simulink model "SimpleImpedance_Main"  (R2016b)
settings: Solver=VariableStepAuto  StartTime=0.0  StopTime=30  RelTol=1e-3  EnableMultiTasking=on
undefined symbols (not defined in the file): b, bh, C, dt, J, Jh, JJ, k, K, K_f, Ke, kh, M
settings Model: Creator=Minsu  LastModifiedBy=Minsu
settings DataIOCC: LimitDataPoints=on
settings OptimizationCC: LifeSpan=inf
settings DebuggingCC: AllowSymbolicDim=off  SFUnexpectedBacktrackingDiag=warning  SFNoUnconditionalDefaultTransitionDiag=warning  SFExecutionAtInitializationDiag=none
settings ModelReferenceCC: PropagateSignalLabelsOutOfModel=off
settings GRTTargetCC: TargetLangStandard=C89/C90 (ANSI)
settings ConfigComp: CovMetricSettings=dw  CovHtmlReporting=on  CovSaveCumulativeToWorkspaceVar=on  CovSaveSingleToWorkspaceVar=on  CovExternalEMLEnable=off

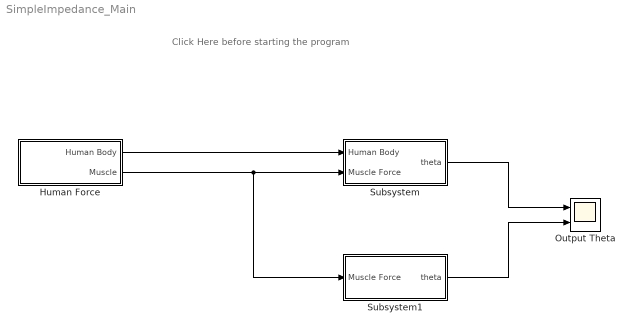
== system SimpleImpedance_Main ==
  note: Click Here before starting the program
  "Human Force " : Subsystem
  Output Theta : Scope  NumInputPorts=2
  Subsystem : Subsystem
  Subsystem1 : Subsystem
  wires:
  "Human Force "/1(Human Body) -> Subsystem/1(Human Body)
  "Human Force "/2(Muscle) -> Subsystem1/1(Muscle Force), Subsystem/2(Muscle Force)
  Subsystem/1(theta) -> Output Theta/1
  Subsystem1/1(theta) -> Output Theta/2

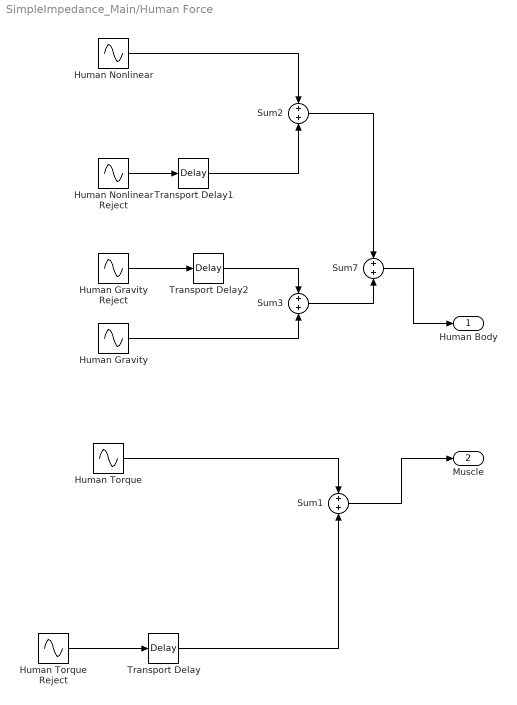
== system SimpleImpedance_Main/Human Force  ==
  Human Gravity : Sin  Amplitude=2  Frequency=2*pi*0.13  Phase=-30*pi/180
  Human Gravity Reject : Sin  Amplitude=-2  Frequency=2*pi*0.13  Phase=-30*pi/180
  Human Nonlinear : Sin  Amplitude=2.1  Frequency=2*pi*1.2
  Human Nonlinear Reject : Sin  Amplitude=-2.1  Frequency=2*pi*1.2
  Human Torque : Sin  Amplitude=10  Frequency=2*JJ*pi
  Human Torque Reject : Sin  Amplitude=-10  Frequency=JJ*2*pi
  Sum{1..3,7} (4 alike) : Sum
  Transport Delay : TransportDelay  DelayTime=3*1/JJ
  Transport Delay1 : TransportDelay  DelayTime=19*1/1.2
  Transport Delay2 : TransportDelay  DelayTime=12*1/0.13
  Human Body : Outport
  Muscle : Outport  Port=2
  wires:
  Sum7/1 -> Human Body/1
  Human Torque Reject/1 -> Transport Delay/1
  Human Torque/1 -> Sum1/1
  Sum1/1 -> Muscle/1
  Transport Delay/1 -> Sum1/2
  Sum2/1 -> Sum7/1
  Sum3/1 -> Sum7/2
  Human Gravity/1 -> Sum3/2
  Human Nonlinear/1 -> Sum2/1
  Human Nonlinear Reject/1 -> Transport Delay1/1
  Transport Delay1/1 -> Sum2/2
  Human Gravity Reject/1 -> Transport Delay2/1
  Transport Delay2/1 -> Sum3/1

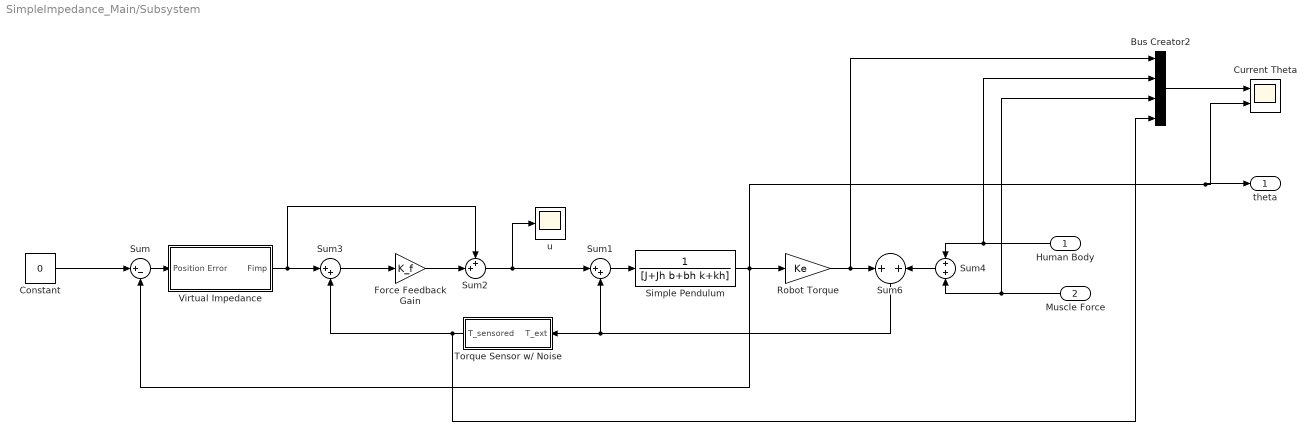
== system SimpleImpedance_Main/Subsystem ==
  Human Body : Inport
  Muscle Force : Inport  Port=2
  Bus Creator2 : BusCreator  Inputs=4
  Constant : Constant  Value=0  SampleTime=dt
  Current Theta : Scope  NumInputPorts=2
  Force Feedback Gain : Gain  Gain=K_f
  Robot Torque : Gain  Gain=Ke
  Simple Pendulum : TransferFcn  Denominator=[J+Jh b+bh k+kh]  ContinuousStateAttributes='Single_Pendulum'
  Sum : Sum  Inputs=|+-
  Sum1 : Sum  Inputs=|++
  Sum2 : Sum  Inputs=++|
  Sum3 : Sum  Inputs=|++
  Sum4 : Sum  Inputs=+|+
  Sum6 : Sum  Inputs=+|+
  Torque Sensor w/ Noise : Subsystem
  Virtual Impedance : Subsystem
  "u " : Scope
  theta : Outport
  wires:
  Sum/1 -> Virtual Impedance/1(Position Error)
  Force Feedback Gain/1 -> Sum2/2
  Sum1/1 -> Simple Pendulum/1
  Sum3/1 -> Force Feedback Gain/1
  Constant/1 -> Sum/1
  Sum2/1 -> Sum1/1, "u "/1
  Muscle Force/1 -> Bus Creator2/3, Sum4/2
  Human Body/1 -> Bus Creator2/2, Sum4/1
  Torque Sensor w/ Noise/1(T_sensored) -> Bus Creator2/4, Sum3/2
  Robot Torque/1 -> Bus Creator2/1, Sum6/1
  Bus Creator2/1 -> Current Theta/1
  Sum4/1 -> Sum6/2
  Sum6/1 -> Sum1/2, Torque Sensor w/ Noise/1(T_ext)
  Simple Pendulum/1 -> theta/1, Current Theta/2, Sum/2, Robot Torque/1
  Virtual Impedance/1(Fimp) -> Sum2/1, Sum3/1

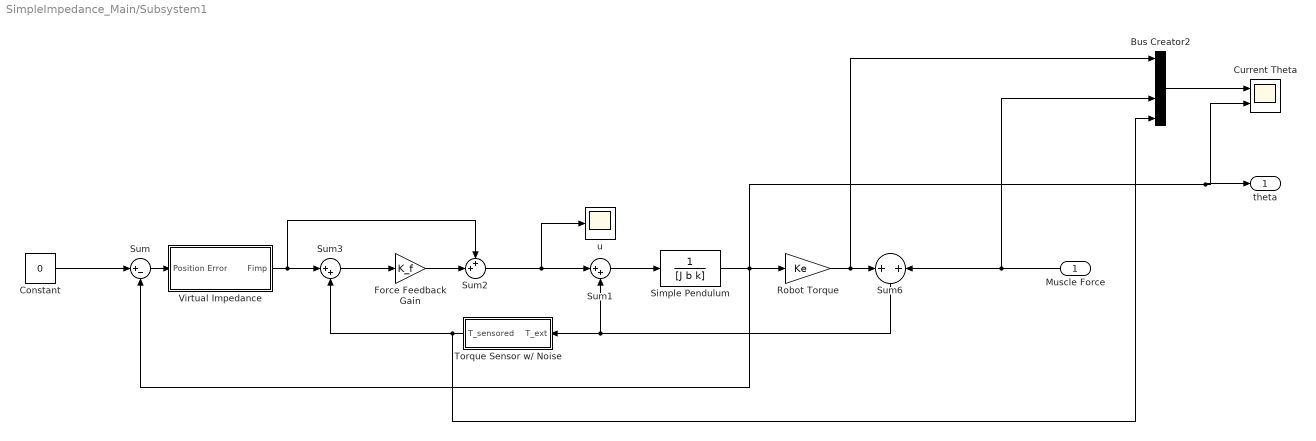
== system SimpleImpedance_Main/Subsystem1 ==
  Muscle Force : Inport
  Bus Creator2 : BusCreator  Inputs=4
  Constant : Constant  Value=0  SampleTime=dt
  Current Theta : Scope  NumInputPorts=2
  Force Feedback Gain : Gain  Gain=K_f
  Robot Torque : Gain  Gain=Ke
  Simple Pendulum : TransferFcn  Denominator=[J b k]  ContinuousStateAttributes='Single_Pendulum'
  Sum : Sum  Inputs=|+-
  Sum1 : Sum  Inputs=|++
  Sum2 : Sum  Inputs=++|
  Sum3 : Sum  Inputs=|++
  Sum6 : Sum  Inputs=+|+
  Torque Sensor w/ Noise : Subsystem
  Virtual Impedance : Subsystem
  "u " : Scope
  theta : Outport
  wires:
  Simple Pendulum/1 -> Robot Torque/1, Sum/2, theta/1, Current Theta/2
  Sum6/1 -> Torque Sensor w/ Noise/1(T_ext), Sum1/2
  Muscle Force/1 -> Sum6/2, Bus Creator2/3
  Bus Creator2/1 -> Current Theta/1
  Robot Torque/1 -> Sum6/1, Bus Creator2/1
  Torque Sensor w/ Noise/1(T_sensored) -> Sum3/2, Bus Creator2/4
  Sum2/1 -> "u "/1, Sum1/1
  Constant/1 -> Sum/1
  Sum3/1 -> Force Feedback Gain/1
  Sum1/1 -> Simple Pendulum/1
  Force Feedback Gain/1 -> Sum2/2
  Virtual Impedance/1(Fimp) -> Sum2/1, Sum3/1
  Sum/1 -> Virtual Impedance/1(Position Error)

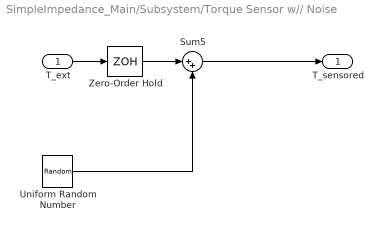
== system SimpleImpedance_Main/Subsystem/Torque Sensor w// Noise ==
  T_ext : Inport
  Sum5 : Sum  Inputs=|++
  Uniform Random Number : UniformRandomNumber  Minimum=-0.5  Maximum=0.5  SampleTime=0.005
  Zero-Order Hold : ZeroOrderHold  SampleTime=dt
  T_sensored : Outport
  wires:
  Zero-Order Hold/1 -> Sum5/1
  T_ext/1 -> Zero-Order Hold/1
  Sum5/1 -> T_sensored/1
  Uniform Random Number/1 -> Sum5/2

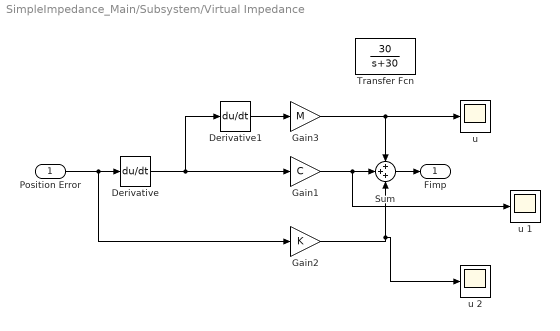
== system SimpleImpedance_Main/Subsystem/Virtual Impedance ==
  Position Error : Inport
  Derivative : Derivative
  Derivative1 : Derivative
  Gain1 : Gain  Gain=C
  Gain2 : Gain  Gain=K
  Gain3 : Gain  Gain=M
  Sum : Sum  Inputs=+++
  Transfer Fcn : TransferFcn  Numerator=[30]  Denominator=[1 30]
  "u " : Scope
  u 1 : Scope
  u 2 : Scope
  Fimp : Outport
  wires:
  Position Error/1 -> Gain2/1, Derivative/1
  Derivative/1 -> Derivative1/1, Gain1/1
  Sum/1 -> Fimp/1
  Derivative1/1 -> Gain3/1
  Gain1/1 -> u 1/1, Sum/2
  Gain3/1 -> "u "/1, Sum/1
  Gain2/1 -> u 2/1, Sum/3

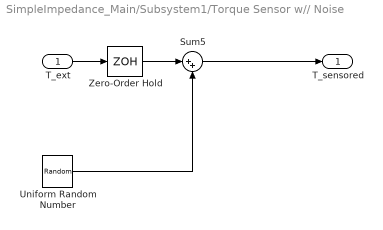
== system SimpleImpedance_Main/Subsystem1/Torque Sensor w// Noise ==
  T_ext : Inport
  Sum5 : Sum  Inputs=|++
  Uniform Random Number : UniformRandomNumber  Minimum=-0.5  Maximum=0.5  SampleTime=0.005
  Zero-Order Hold : ZeroOrderHold  SampleTime=dt
  T_sensored : Outport
  wires:
  Uniform Random Number/1 -> Sum5/2
  Sum5/1 -> T_sensored/1
  T_ext/1 -> Zero-Order Hold/1
  Zero-Order Hold/1 -> Sum5/1

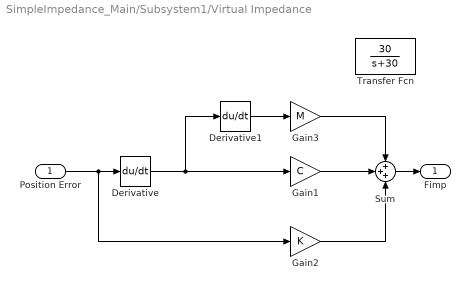
== system SimpleImpedance_Main/Subsystem1/Virtual Impedance ==
  Position Error : Inport
  Derivative : Derivative
  Derivative1 : Derivative
  Gain1 : Gain  Gain=C
  Gain2 : Gain  Gain=K
  Gain3 : Gain  Gain=M
  Sum : Sum  Inputs=+++
  Transfer Fcn : TransferFcn  Numerator=[30]  Denominator=[1 30]
  Fimp : Outport
  wires:
  Gain3/1 -> Sum/1
  Gain2/1 -> Sum/3
  Gain1/1 -> Sum/2
  Derivative1/1 -> Gain3/1
  Sum/1 -> Fimp/1
  Derivative/1 -> Gain1/1, Derivative1/1
  Position Error/1 -> Derivative/1, Gain2/1
